simulink model "iddempr2"  (R2016a)
settings: Solver=ode45  StartTime=0.0  StopTime=500  RelTol=1e-3
settings Model: ExtModeTrigMode=oneshot  ExtModeArmWhenConnect=off  ExtModeAutoUpdateStatusClock=off  Creator=The MathWorks, Inc.  LastModifiedBy=The MathWorks, Inc.
settings DataIOCC: SaveFormat=Array
settings OptimizationCC: BooleanDataType=off  InitFltsAndDblsToZero=on
settings DebuggingCC: SaveWithParameterizedLinksMsg=none  UnderspecifiedInitializationDetection=Classic  MergeDetectMultiDrivingBlocksExec=none  SignalResolutionControl=TryResolveAllWithWarning  MultiTaskDSMMsg=warning  MultiTaskCondExecSysMsg=none  IntegerOverflowMsg=none  FcnCallInpInsideContextMsg=UseLocalSettings  StrictBusMsg=None  IntegerSaturationMsg=none
settings HardwareCC: ProdBitPerPointer=32  ProdLargestAtomicFloat=None  ProdIntDivRoundTo=Undefined  ProdEndianess=Unspecified  ProdWordSize=32  ProdHWDeviceType=32-bit Generic  TargetUnknown=on
settings ModelReferenceCC: PropagateSignalLabelsOutOfModel=off
settings GRTTargetCC: TargetFcnLib=ansi_tfl_tmw.mat  GeneratePreprocessorConditionals=Use local settings  CombineOutputUpdateFcns=off  GRTInterface=on
settings ConfigComp: CovModelRefEnable=Off

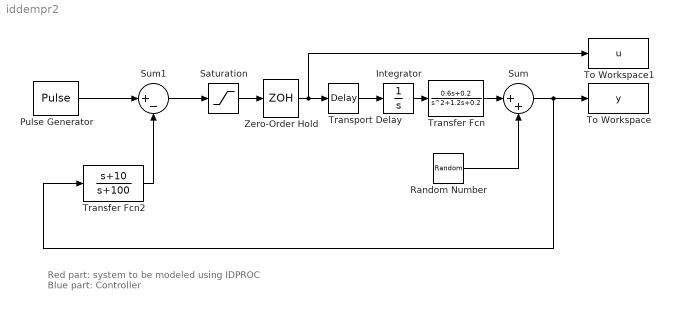
== system iddempr2 ==
  note: Red part: system to be modeled using IDPROC
      | Blue part: Controller
  Integrator : Integrator
  Pulse Generator : DiscretePulseGenerator  Period=200  PulseWidth=50
  Random Number : RandomNumber  Variance=0.1  SampleTime=1
  Saturation : Saturate
  Sum : Sum  Inputs=|++  SaturateOnIntegerOverflow=on  InputSameDT=on  OutDataTypeStr=Inherit: Same as first input
  Sum1 : Sum  Inputs=|+-  SaturateOnIntegerOverflow=on  InputSameDT=on  OutDataTypeStr=Inherit: Same as first input
  To Workspace : ToWorkspace  VariableName=y  SampleTime=1
  To Workspace1 : ToWorkspace  VariableName=u  SampleTime=1
  Transfer Fcn : TransferFcn  Numerator=[0.6 0.2]  Denominator="[1 1.2  0.2]"
  Transfer Fcn2 : TransferFcn  Numerator=[1 10]  Denominator=[1 100]
  Transport Delay : TransportDelay  DelayTime=2.2
  Zero-Order Hold : ZeroOrderHold
  wires:
  Transfer Fcn/1 -> Sum/1
  Random Number/1 -> Sum/2
  Sum/1 -> To Workspace/1, Transfer Fcn2/1
  Zero-Order Hold/1 -> To Workspace1/1, Transport Delay/1
  Transport Delay/1 -> Integrator/1
  Integrator/1 -> Transfer Fcn/1
  Sum1/1 -> Saturation/1
  Saturation/1 -> Zero-Order Hold/1
  Transfer Fcn2/1 -> Sum1/2
  Pulse Generator/1 -> Sum1/1
